simulink model "pi_sim_2022b"  (R2023b)
settings: Solver=ode45  StartTime=0.0  StopTime=1200  FixedStep=0.1  RelTol=1e-3  EnableMultiTasking=on
undefined symbols (not defined in the file or in its folder): Advantech, PCI
libraries: sldrtlib x4, SignalEditorBlockLib x2
settings Model: Creator=Admin  LastModifiedBy=andre
settings SolverCC: AlgebraicLoopSolver=TrustRegion
settings DataIOCC: LimitDataPoints=on  SaveFormat=Array  ReturnWorkspaceOutputs=off
settings OptimizationCC: ReuseModelBlockBuffer=off  LifeSpan=inf
settings DebuggingCC: UnconnectedInputMsg=warning  UnconnectedOutputMsg=warning  UnconnectedLineMsg=warning  SFUnexpectedBacktrackingDiag=warning  SFNoUnconditionalDefaultTransitionDiag=warning  SFExecutionAtInitializationDiag=none  ArithmeticOperatorsInVariantConditions=warning
settings HardwareCC: ProdBitPerPointer=32  ProdBitPerSizeT=32  ProdBitPerPtrDiffT=32  ProdLargestAtomicFloat=None  ProdIntDivRoundTo=Undefined  ProdEndianess=Unspecified  ProdWordSize=32  ProdHWDeviceType=32-bit Generic
settings ModelReferenceCC: PropagateSignalLabelsOutOfModel=off
settings SFSimCC: SimUseLocalCustomCode=off  CustomCodeUndefinedFunction=UseInterfaceOnly
settings RTWCC: RTWUseLocalCustomCode=off
settings CodeAppCC: StateflowObjectComments=on
settings GRTTargetCC: TargetLangStandard=C89/C90 (ANSI)
settings ConfigComp: CovMetricSettings=dw  CovSaveCumulativeToWorkspaceVar=on  CovSaveSingleToWorkspaceVar=on  CovExternalEMLEnable=off

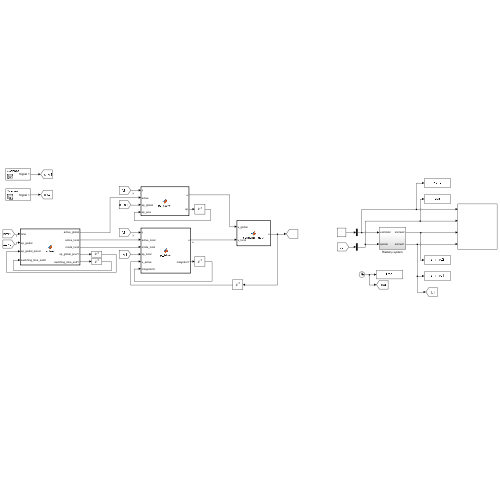
[thumbnail: Simulink's stored preview of the top-level diagram]
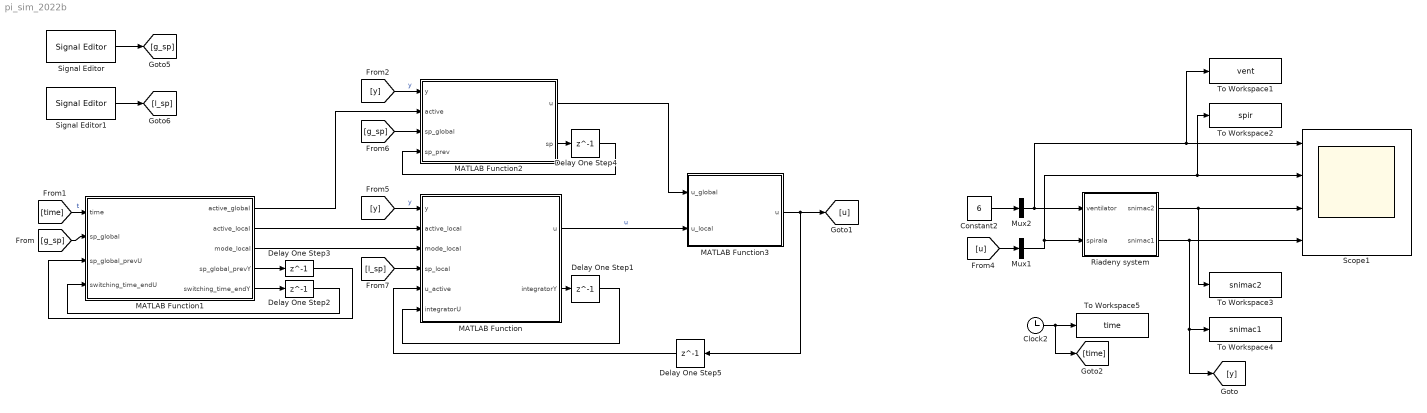
== system pi_sim_2022b ==
  Clock2 : Clock
  Constant2 : Constant  Value=6
  Delay One Step{1..5} (5 alike) : Delay  DelayLength=1
  MATLAB Function : MATLAB Function  TreatAsAtomicUnit=on
  MATLAB Function1 : MATLAB Function  TreatAsAtomicUnit=on
  MATLAB Function2 : MATLAB Function  TreatAsAtomicUnit=on
  MATLAB Function3 : MATLAB Function  TreatAsAtomicUnit=on
  Mux1 : Mux  Inputs=1
  Mux2 : Mux  Inputs=1
  Riadeny system : Subsystem
  Scope1 : Scope  NumInputPorts=4
  Signal Editor : SignalEditorBlockLib/Signal Editor  FileName=C:\MyFiles\Study\DP-Stoliar\ML\TS\PID\PI_switch_forPBs\global_sp.mat  ActiveScenario=Scenario  ActiveSignal=Signal 1  IsBus=off  OutputBusObjectStr=Bus: BusObject  SampleTime=0  Interpolate=off  ZeroCross=off  OutputAfterFinalValue=Setting to zero  Unit=inherit  PreserveSignalName=on  ApplySigPropsToAllScenarios=on  ApplySigPropsToAllSignals=off
  Signal Editor1 : SignalEditorBlockLib/Signal Editor  FileName=C:\MyFiles\Study\DP-Stoliar\ML\TS\PID\PI_switch_forPBs\local_sp.mat  ActiveScenario=Scenario  ActiveSignal=Signal 1  IsBus=off  OutputBusObjectStr=Bus: BusObject  SampleTime=0  Interpolate=off  ZeroCross=off  OutputAfterFinalValue=Setting to zero  Unit=inherit  PreserveSignalName=on  ApplySigPropsToAllScenarios=on  ApplySigPropsToAllSignals=off
  To Workspace1 : ToWorkspace  VariableName=vent  SampleTime=0.1
      settings: Save2DSignal=2-D array (concatenate along first dimension)
  To Workspace2 : ToWorkspace  VariableName=spir  SampleTime=0.1
      settings: Save2DSignal=2-D array (concatenate along first dimension)
  To Workspace3 : ToWorkspace  VariableName=snimac2  SampleTime=0.1
      settings: Save2DSignal=2-D array (concatenate along first dimension)
  To Workspace4 : ToWorkspace  VariableName=snimac1  SampleTime=0.1
      settings: Save2DSignal=2-D array (concatenate along first dimension)
  To Workspace5 : ToWorkspace  VariableName=time  SampleTime=0.1
      settings: Save2DSignal=2-D array (concatenate along first dimension)
  wires:
  [y] -> MATLAB Function/1(y)  "y"
  [u] -> Mux1/1
  Mux1/1 -> Riadeny system/2(spirala), To Workspace2/1, Scope1/2
  Riadeny system/2(snimac1) -> [y], To Workspace4/1, Scope1/4
  Mux2/1 -> Riadeny system/1(ventilator), To Workspace1/1, Scope1/1
  Riadeny system/1(snimac2) -> To Workspace3/1, Scope1/3
  Clock2/1 -> [time], To Workspace5/1
  Constant2/1 -> Mux2/1
  [time] -> MATLAB Function1/1(time)  "t"
  MATLAB Function1/4(sp_global_prevY) -> Delay One Step3/1
  MATLAB Function1/5(switching_time_endY) -> Delay One Step2/1
  Delay One Step2/1 -> MATLAB Function1/4(switching_time_endU)
  Delay One Step3/1 -> MATLAB Function1/3(sp_global_prevU)
  MATLAB Function1/1(active_global) -> MATLAB Function2/2(active)
  MATLAB Function2/2(sp) -> Delay One Step4/1
  [y] -> MATLAB Function2/1(y)  "y"
  Delay One Step4/1 -> MATLAB Function2/4(sp_prev)
  MATLAB Function1/2(active_local) -> MATLAB Function/2(active_local)
  MATLAB Function/2(integratorY) -> Delay One Step1/1
  Delay One Step1/1 -> MATLAB Function/6(integratorU)
  MATLAB Function2/1(u) -> MATLAB Function3/1(u_global)
  MATLAB Function/1(u) -> MATLAB Function3/2(u_local)  "u"
  MATLAB Function3/1(u) -> [u], Delay One Step5/1
  Signal Editor1/1 -> [l_sp]
  Signal Editor/1 -> [g_sp]
  [g_sp] -> MATLAB Function1/2(sp_global)
  [g_sp] -> MATLAB Function2/3(sp_global)
  [l_sp] -> MATLAB Function/4(sp_local)
  Delay One Step5/1 -> MATLAB Function/5(u_active)
  MATLAB Function1/3(mode_local) -> MATLAB Function/3(mode_local)

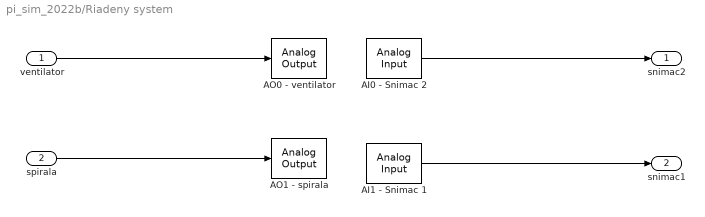
== system pi_sim_2022b/Riadeny system ==
  ventilator : Inport
  spirala : Inport  Port=2
  AI0 - Snimac 2 : sldrtlib/Analog Input  SampleTime=0.1  MaxMissedTicks=10  ShowMissedTicks=off  YieldWhenWaiting=off  DrvName=Advantech/PCI-1711  DrvAddress=4294967295  DrvOptions=zeros(1,0)  Channels=1  RangeMode=1  VoltRange=1  DataType=1
      settings: AttributesFormatString=Advantech\nPCI-1711 [auto]
  AI1 - Snimac 1 : sldrtlib/Analog Input  SampleTime=0.1  MaxMissedTicks=10  ShowMissedTicks=off  YieldWhenWaiting=off  DrvName=Advantech/PCI-1711  DrvAddress=4294967295  DrvOptions=zeros(1,0)  Channels=2  RangeMode=1  VoltRange=1  DataType=1
      settings: AttributesFormatString=Advantech\nPCI-1711 [auto]
  AO0 - ventilator : sldrtlib/Analog Output  SampleTime=0.1  MaxMissedTicks=10  ShowMissedTicks=off  YieldWhenWaiting=off  DrvName=Advantech/PCI-1711  DrvAddress=4294967295  DrvOptions=zeros(1,0)  Channels=1  RangeMode=1  VoltRange=2  InitialValue=[]  FinalValue=[]
      settings: AttributesFormatString=Advantech\nPCI-1711 [auto]
  AO1 - spirala : sldrtlib/Analog Output  SampleTime=0.1  MaxMissedTicks=10  ShowMissedTicks=off  YieldWhenWaiting=off  DrvName=Advantech/PCI-1711  DrvAddress=4294967295  DrvOptions=zeros(1,0)  Channels=2  RangeMode=1  VoltRange=2  InitialValue=[]  FinalValue=[]
      settings: AttributesFormatString=Advantech\nPCI-1711 [auto]
  snimac2 : Outport
  snimac1 : Outport  Port=2
  wires:
  ventilator/1 -> AO0 - ventilator/1
  spirala/1 -> AO1 - spirala/1
  AI1 - Snimac 1/1 -> snimac1/1
  AI0 - Snimac 2/1 -> snimac2/1

== matlab function pi_sim_2022b/MATLAB Function1 ==
  data: active_global output; time input; sp_global input; sp_global_prevU input; active_local output; mode_local output; switching_time_endU input; sp_global_prevY output; switching_time_endY output
function [active_global, active_local, mode_local, sp_global_prevY, switching_time_endY]  = solver(time, sp_global, sp_global_prevU, switching_time_endU)

    %Constants
    step_to_soft = 0.005;
    Ts = 0.1;
    extra_time = 10;
    esp = 1e-5;

    active_global = 0;
    active_local = 0;

    %Time of switch working
    if abs(sp_global - sp_global_prevU) > eps
        reg_time = (abs(sp_global - sp_global_prevU) / step_to_soft) * Ts + extra_time;
        reg_time = max(reg_time, extra_time);
        switching_time_endY = time + reg_time;
    else
        switching_time_endY = switching_time_endU;
    end

    %Activators of PI and switch
    if time < switching_time_endY
        active_global = 1;
        active_local = 0;
    else
        active_global = 0;
        active_local = 1;
    end

    if sp_global > 7.6
        mode_local = 6;
    elseif sp_global > 6.2
        mode_local = 4;
    else
        mode_local = 2;
    end

    %memory 
    sp_global_prevY = sp_global;
       
end

== matlab function pi_sim_2022b/MATLAB Function ==
  data: y input; active_local input; mode_local input; u output; sp_local input; u_active input; integratorY output; integratorU input
function [u, integratorY] = pi_block(y, active_local, mode_local, sp_local, u_active, integratorU)

    Ts = 0.1;
    
    %Gain scheduling
    
    if mode_local == 2
        pb_u = 2; pb_y = 4.4884;
        Kp = 2.77; Ki = 1.48;
    elseif mode_local == 4
        pb_u = 4; pb_y = 6.3412;
        Kp = 3.58; Ki = 1.84;
    else
        pb_u = 6; pb_y = 7.7441;
        Kp = 1.83; Ki = 2.20;
    end
    
    u_min = 0 - pb_u;
    u_max = 10 - pb_u;
    
    yN = y - pb_y;
    
    e = sp_local - yN;
 
    if active_local == 0
        uN = u_active - pb_u;
        uN = min(max(uN, u_min), u_max);
        integratorY = (uN - Kp*e)/ Ki;
        u = 0;
    else
        integratorY = integratorU + e*Ts;
        uN = Kp*e + Ki*integratorY;
        uN = min(max(uN, u_min), u_max);
        u = uN + pb_u;
    end

end

== matlab function pi_sim_2022b/MATLAB Function2 ==
  data: y input; u output; sp output; active input; sp_global input; sp_prev input
function [u, sp] = pb_switch(y, active, sp_global, sp_prev)

%Constants

Kp = 4;
Ts = 0.1;
step_to_soft = 0.005;

%Logic

if active

    if abs(sp_global - sp_prev) > step_to_soft
        delta = sign(sp_global - sp_prev) * step_to_soft;
    else
        delta = sp_global - sp_prev;
    end

    sp = sp_prev + delta;
    u = Kp * (sp-y);

else

    sp = sp_global;
    u = 0;

end

    u = min(max(u,0), 10);
    
end

== matlab function pi_sim_2022b/MATLAB Function3 ==
  data: u_global input; u output; u_local input
function u = normalize_input(u_global, u_local)

    u_sum = u_global + u_local;
    
    u = min(max(u_sum, 0), 10);

end
